simulink model "pll"  (Simulink 7.9)
settings: Solver=ode45  StartTime=0.0  StopTime=.05  RelTol=1e-3
undefined symbols (not defined in the file or in its folder): dfilt
libraries: dsparch4 x1, commsynccomp2 x1, dspsrcs4 x1
settings Model: Creator=ArunKB  LastModifiedBy=ArunKB

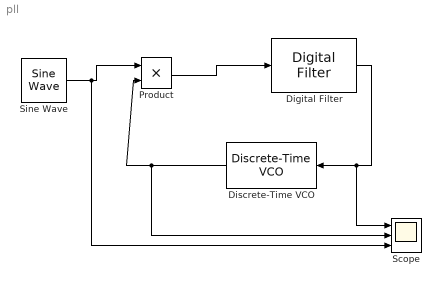
== system pll ==
  Digital Filter : dsparch4/Digital Filter  TypePopup=FIR (all zeros)  IIRFiltStruct=Direct form II transposed  AllPoleFiltStruct=Direct form  FIRFiltStruct=Direct form  CoeffSource=Specify via dialog  NumCoeffs=k  DenCoeffs=[1 0.1]  BiQuadCoeffs=[1 0.3 0.4 1 0.1 0.2]  LatticeCoeffs=[0.2 0.4]  denIgnore=on  FiltPerSampPopup=One filter per frame  IC=0  ICnum=0  ICden=0  roundingMode=Floor  overflowMode=off  ScaleValues=1  scaleValueFracLength=14  stageInFracLength=15  stageOutFracLength=15  FilterSource=Specify via dialog  dfiltObjectName=dfilt.dffir([1 2 1])  InputProcessing=Columns as channels (frame based)
  Discrete-Time VCO : commsynccomp2/Discrete-Time VCO  Ac=1  Fc=2000  Kc=1  Ph=-pi  ts=1/96000
  Product : Product  RndMeth=Zero
  Scope : Scope  NumInputPorts=3
      settings: TickLabels=on  TimeRange=0.01  YMin=-5~-1~-5  YMax=5~1~5  SampleInput=on
  Sine Wave : dspsrcs4/Sine Wave  Amplitude=1  Frequency=2000  Phase=pi  SampleMode=Discrete  OutComplex=Real  CompMethod=Table lookup  TableSize=Speed  SampleTime=1/96000  SamplesPerFrame=1  ResetState=Restart at time zero  dataType=double  wordLen=16  udDataType=sfix(16)  fracBitsMode=Best precision  numFracBits=15  OutDataTypeStr=double  LastOutDataTypeStr=double
  wires:
  Sine Wave/1 -> Product/1, Scope/3
  Discrete-Time VCO/1 -> Product/2, Scope/2
  Product/1 -> Digital Filter/1
  Digital Filter/1 -> Discrete-Time VCO/1, Scope/1
